simulink model "Simulation_WTA"  (R2020b)
settings: Solver=ode45  StartTime=0.0  StopTime=100  RelTol=1e-3  EnableMultiTasking=on
InitFcn:
  | n = 7
(part 1 of 4)
settings Model: Creator=LVQ  LastModifiedBy=levie
settings DataIOCC: LimitDataPoints=on  SaveFormat=Array  ReturnWorkspaceOutputs=off
settings OptimizationCC: LifeSpan=inf
settings DebuggingCC: SolverPrmCheckMsg=warning  SFUnexpectedBacktrackingDiag=warning  SFNoUnconditionalDefaultTransitionDiag=warning  SFExecutionAtInitializationDiag=none  ArithmeticOperatorsInVariantConditions=warning
settings HardwareCC: ProdBitPerPointer=32  ProdBitPerSizeT=32  ProdBitPerPtrDiffT=32  ProdLargestAtomicFloat=None  ProdIntDivRoundTo=Undefined  ProdEndianess=Unspecified  ProdWordSize=32  ProdHWDeviceType=32-bit Generic
settings ModelReferenceCC: PropagateSignalLabelsOutOfModel=off
settings SFSimCC: SimUseLocalCustomCode=off  CustomCodeUndefinedFunction=UseInterfaceOnly
settings RTWCC: RTWUseLocalCustomCode=off
settings CodeAppCC: StateflowObjectComments=on
settings GRTTargetCC: TargetLangStandard=C89/C90 (ANSI)
settings ConfigComp: CovMetricSettings=dw  CovSaveCumulativeToWorkspaceVar=on  CovSaveSingleToWorkspaceVar=on  CovExternalEMLEnable=off  CovSFcnEnable=off

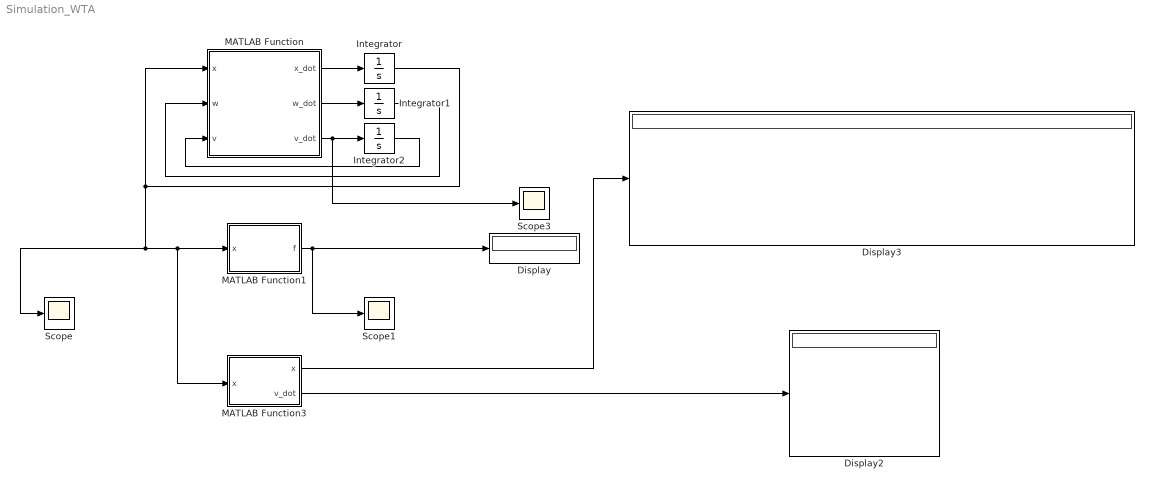
== system Simulation_WTA ==
  Display : Display
  Display2 : Display
  Display3 : Display
  Integrator : Integrator  InitialCondition=zeros(n*n,1)
  Integrator1 : Integrator  InitialCondition=ones(n*n,1)
  Integrator2 : Integrator  InitialCondition=ones(2*n,1)
  MATLAB Function : MATLAB Function  TreatAsAtomicUnit=on
  MATLAB Function1 : MATLAB Function  TreatAsAtomicUnit=on
  MATLAB Function3 : MATLAB Function  TreatAsAtomicUnit=on
  Scope : Scope
  Scope1 : Scope
  Scope3 : Scope
  wires:
  MATLAB Function/1(x_dot) -> Integrator/1
  MATLAB Function/2(w_dot) -> Integrator1/1
  MATLAB Function/3(v_dot) -> Scope3/1, Integrator2/1
  Integrator/1 -> Scope/1, MATLAB Function3/1("x "), MATLAB Function1/1(x), MATLAB Function/1(x)
  Integrator1/1 -> MATLAB Function/2(w)
  Integrator2/1 -> MATLAB Function/3(v)
  MATLAB Function1/1(f) -> Scope1/1, Display/1
  MATLAB Function3/2(v_dot) -> Display2/1
  MATLAB Function3/1(x) -> Display3/1
